simulink model "GraphFun1NoActions"  (Simulink 9.0)
settings: Solver=FixedStepDiscrete  StartTime=0.0  StopTime=19.8  FixedStep=0.200000  RelTol=1e-3  EnableMultiTasking=on
model workspace (MAT data in the model file):
  already_pp = 1
  input_dataset = Simulink.SimulationData.Dataset
  input_dataset.any.Name = ''
  input_dataset.any.Version = 3
  input_dataset.any.Storage = Simulink.SimulationData.Storage.RamDatasetStorage
  input_dataset.any.Storage.any.Version = 2
  input_dataset.any.Storage.any.Elements{1} = Simulink.SimulationData.Signal
  input_dataset.any.Storage.any.Elements{1}.Version = 1
  input_dataset.any.Storage.any.Elements{1}.Values = timeseries
  input_dataset.any.Storage.any.Elements{1}.Values.Name = 'unnamed'
  input_dataset.any.Storage.any.Elements{1}.Values.DataInfo = tsdata.datametadata
  input_dataset.any.Storage.any.Elements{1}.Values.DataInfo.Interpolation = tsdata.interpolation
  input_dataset.any.Storage.any.Elements{1}.Values.DataInfo.Interpolation.Fhandle : function handle (value not decoded)
  input_dataset.any.Storage.any.Elements{1}.Values.DataInfo.Interpolation.Name = 'linear'
  input_dataset.any.Storage.any.Elements{1}.Values.TimeInfo = tsdata.timemetadata
  input_dataset.any.Storage.any.Elements{1}.Values.TimeInfo.Length = 100
  input_dataset.any.Storage.any.Elements{1}.Values.TimeInfo.DuplicateTimes = 0
  input_dataset.any.Storage.any.Elements{1}.Values.TimeInfo.Time_ = [0; 0.2; 0.4; 0.6; 0.8; 1; 1.2; 1.4; 1.6; 1.8; 2; 2.2; 2.4; 2.6; 2.8; 3; 3.2; 3.4; 3.6; 3.8; 4; 4.2; 4.4; 4.6; 4.8; 5; 5.2; 5.4; 5.6; 5.8; 6; 6.2; 6.4; 6.6; 6.8; 7; 7.2; 7.4; 7.6; 7.8; 8; 8.2; 8.4; 8.6; 8.8; 9; 9.2; 9.4; 9.6; 9.8; 10; 10.2; 10.4; 10.6; 10.8; 11; 11.2; 11.4; 11.6; 11.8; 12; 12.2; 12.4; 12.6; 12.8; 13; 13.2; 13.4; 13.6; 13.8; 14; 14.2; 14.4; 14.6; 14.8; 15; 15.2; 15.4; 15.6; 15.8; 16; 16.2; 16.4; 16.6; 16.8; 17; 17.2; 17.4; 17.6; 17.8; 18; 18.2; 18.4; 18.6; 18.8; 19; 19.2; 19.4; 19.6; 19.8]
  input_dataset.any.Storage.any.Elements{1}.Values.TimeInfo.Initialized = 1
  input_dataset.any.Storage.any.Elements{1}.Values.QualityInfo = tsdata.qualmetadata
  input_dataset.any.Storage.any.Elements{1}.Values.Data_ = [1; 1; 1; 1; 0; 0; 0; 1; 1; 1; 1; 0; 1; 1; 0; 1; 1; 0; 1; 1; 0; 0; 0; 1; 1; 0; 1; 1; 1; 1; 0; 0; 1; 0; 0; 0; 1; 0; 1; 0; 1; 0; 0; 1; 0; 1; 1; 0; 0; 0; 0; 0; 1; 1; 1; 1; 0; 1; 0; 1; 0; 1; 0; 1; 1; 1; 1; 1; 0; 0; 1; 1; 1; 0; 1; 1; 0; 1; 1; 0; 1; 1; 0; 1; 1; 1; 1; 0; 0; 1; 1; 0; 0; 0; 0; 0; 1; 0; 0; 0]
  input_dataset.any.Storage.any.Elements{1}.Name = 'In1'
  input_dataset.any.Storage.any.Elements{2} = Simulink.SimulationData.Signal
  input_dataset.any.Storage.any.Elements{2}.Version = 1
  input_dataset.any.Storage.any.Elements{2}.Values = timeseries
  input_dataset.any.Storage.any.Elements{2}.Values.Name = 'unnamed'
  input_dataset.any.Storage.any.Elements{2}.Values.DataInfo = tsdata.datametadata
  input_dataset.any.Storage.any.Elements{2}.Values.DataInfo.Interpolation = tsdata.interpolation
  input_dataset.any.Storage.any.Elements{2}.Values.DataInfo.Interpolation.Fhandle : function handle (value not decoded)
  input_dataset.any.Storage.any.Elements{2}.Values.DataInfo.Interpolation.Name = 'linear'
  input_dataset.any.Storage.any.Elements{2}.Values.TimeInfo = tsdata.timemetadata
  input_dataset.any.Storage.any.Elements{2}.Values.TimeInfo.Length = 100
  input_dataset.any.Storage.any.Elements{2}.Values.TimeInfo.DuplicateTimes = 0
  input_dataset.any.Storage.any.Elements{2}.Values.TimeInfo.Time_ = [0; 0.2; 0.4; 0.6; 0.8; 1; 1.2; 1.4; 1.6; 1.8; 2; 2.2; 2.4; 2.6; 2.8; 3; 3.2; 3.4; 3.6; 3.8; 4; 4.2; 4.4; 4.6; 4.8; 5; 5.2; 5.4; 5.6; 5.8; 6; 6.2; 6.4; 6.6; 6.8; 7; 7.2; 7.4; 7.6; 7.8; 8; 8.2; 8.4; 8.6; 8.8; 9; 9.2; 9.4; 9.6; 9.8; 10; 10.2; 10.4; 10.6; 10.8; 11; 11.2; 11.4; 11.6; 11.8; 12; 12.2; 12.4; 12.6; 12.8; 13; 13.2; 13.4; 13.6; 13.8; 14; 14.2; 14.4; 14.6; 14.8; 15; 15.2; 15.4; 15.6; 15.8; 16; 16.2; 16.4; 16.6; 16.8; 17; 17.2; 17.4; 17.6; 17.8; 18; 18.2; 18.4; 18.6; 18.8; 19; 19.2; 19.4; 19.6; 19.8]
  input_dataset.any.Storage.any.Elements{2}.Values.TimeInfo.Initialized = 1
  input_dataset.any.Storage.any.Elements{2}.Values.QualityInfo = tsdata.qualmetadata
  input_dataset.any.Storage.any.Elements{2}.Values.Data_ = [0; 0; 0; 0; 0; 0; 0; 0; 0; 1; 0; 1; 0; 0; 0; 0; 0; 0; 0; 0; 0; 0; 1; 1; 1; 0; 0; 0; 1; 0; 0; 0; 0; 0; 1; 0; 1; 1; 0; 1; 1; 1; 1; 0; 1; 0; 0; 1; 1; 0; 0; 1; 1; 1; 1; 0; 1; 0; 1; 0; 1; 1; 0; 0; 0; 0; 0; 1; 0; 1; 0; 0; 0; 0; 1; 1; 1; 1; 0; 0; 0; 0; 0; 1; 1; 1; 0; 0; 1; 1; 1; 1; 1; 1; 0; 1; 0; 0; 0; 0]
  input_dataset.any.Storage.any.Elements{2}.Name = 'In2'
settings Model: SuppressorTable=22 serialization::archive 11 0 6 0 0 0 0 0  Creator=scaife  LastModifiedBy=hbourbou  ExtModeAutoUpdateStatusClock=off
settings DataIOCC: ExternalInput=input_dataset  LimitDataPoints=on  LoadExternalInput=on  SaveFormat=Dataset  SignalLoggingSaveFormat=ModelDataLogs  SaveState=on
settings OptimizationCC: InitFltsAndDblsToZero=on
settings DebuggingCC: AlgebraicLoopMsg=error  ArtificialAlgebraicLoopMsg=error  SaveWithParameterizedLinksMsg=none  SignalResolutionControl=TryResolveAllWithWarning  SolverPrmCheckMsg=warning  MultiTaskDSMMsg=warning  MultiTaskCondExecSysMsg=none  SingleTaskRateTransMsg=error
settings SFSimCC: SimParseCustomCode=off
settings GRTTargetCC: TargetFcnLib=ansi_tfl_tmw.mat  CombineOutputUpdateFcns=off  GRTInterface=on  ExtMode=on

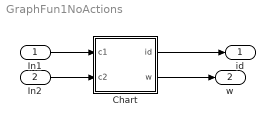
== system GraphFun1NoActions ==
  In1 : Inport  OutDataTypeStr=boolean
  In2 : Inport  Port=2  OutDataTypeStr=boolean
  Chart : Stateflow chart  TreatAsAtomicUnit=on
  id : Outport
  w : Outport  Port=2
  wires:
  Chart/1(id) -> id/1
  In1/1 -> Chart/1(c1)
  In2/1 -> Chart/2(c2)
  Chart/2(w) -> w/1

== stateflow chart Chart ==
  state A/
    en:[id, w]=f(1.0,int32(1));
  state B/
    en:[id, w]=f(2,int32(2));
  state [z1, z2]=f(x,y) [function]
    (default) -> (junction 11) : {z1=x*x;}
    (junction 11) -> (junction 10) : {z2 = 3.0;}
  (default) -> A
  A -> B : [c1]
  B -> A : [c2]
  data: x function_input double; y function_input int32; z1 function_output double; z2 function_output double; c1 input boolean; c2 input boolean; id output double; w output double
